simulink model "TCPZybo"  (Simulink 8.3)
settings: Solver=FixedStepDiscrete  StartTime=0.0  StopTime=inf  FixedStep=0.5  RelTol=1e-3
StartFcn:
  | localAddEventListener
libraries: simulink x5, hdlsllib x2, instrumentlib x2
settings Model: xpc_rtwmakecfg_data=_xpcetherlib__xpcether8255xlib__xpcetherGbElib__xpcnblib_  Creator=laca  LastModifiedBy=laca
settings OptimizationCC: BlockReduction=off
settings DebuggingCC: UnderspecifiedInitializationDetection=Simplified  MultiTaskDSMMsg=warning  MultiTaskCondExecSysMsg=none  StateNameClashWarn=none
settings RTWCC: IncludeERTFirstTime=on
settings GRTTargetCC: CombineOutputUpdateFcns=on  GRTInterface=off

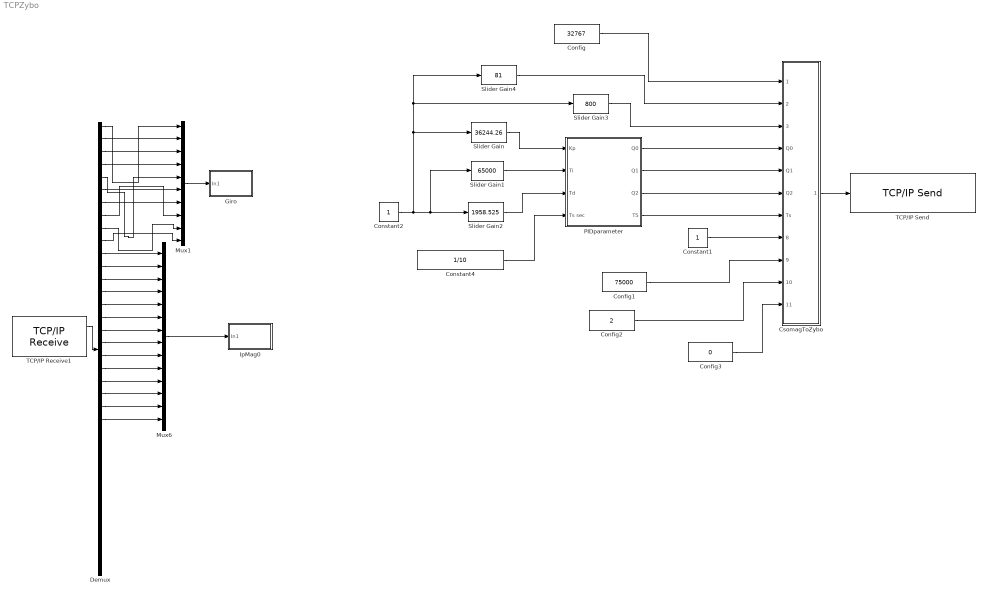
== system TCPZybo ==
  Config : Constant  Value=32767
  Config1 : Constant  Value=75000
  Config2 : Constant  Value=2
  Config3 : Constant  Value=0
  Constant1 : Constant
  Constant2 : Constant
  Constant4 : Constant  Value=1/10
  CsomagToZybo : Subsystem
  Demux : Demux  Outputs=36
  Giro : Subsystem
  IpMag0 : Subsystem
  Mux1 : Mux  Inputs=10
  Mux6 : Mux  Inputs=14
  PIDparameter : Subsystem
  Slider Gain : simulink/Math Operations/Slider Gain  low=0  gain=36244.26  high=65000
  Slider Gain1 : simulink/Math Operations/Slider Gain  low=0  gain=65000  high=65000
  Slider Gain2 : simulink/Math Operations/Slider Gain  low=0  gain=1958.525  high=5000
  Slider Gain3 : simulink/Math Operations/Slider Gain  low=-10000  gain=800  high=10000
  Slider Gain4 : simulink/Math Operations/Slider Gain  low=-180  gain=81  high=180
  TCP/IP Receive1 : instrumentlib/TCP//IP Receive  Host=192.168.0.10  Port=7  DataSize="[1  36]"  EnableBlockingMode=off  Timeout=100  SampleTime=1  DataType=int16  ByteOrder=LittleEndian
  TCP/IP Send : instrumentlib/TCP//IP Send  Host=192.168.0.10  Port=7  EnableBlockingMode=off  Timeout=10  ByteOrder=LittleEndian
  wires:
  Demux/1 -> Mux1/1
  Demux/2 -> Mux1/2
  Demux/3 -> Mux1/3
  TCP/IP Receive1/1 -> Demux/1
  Demux/11 -> Mux6/1
  Demux/24 -> Mux6/14
  Demux/23 -> Mux6/13
  Demux/22 -> Mux6/12
  Demux/21 -> Mux6/11
  Demux/20 -> Mux6/10
  Demux/19 -> Mux6/9
  Demux/18 -> Mux6/8
  Demux/17 -> Mux6/7
  Demux/16 -> Mux6/6
  Demux/15 -> Mux6/5
  Demux/14 -> Mux6/4
  Demux/13 -> Mux6/3
  Demux/12 -> Mux6/2
  Mux6/1 -> IpMag0/1(In1)
  Demux/10 -> Mux1/10
  Demux/9 -> Mux1/9
  Demux/8 -> Mux1/8
  Demux/7 -> Mux1/7
  Demux/6 -> Mux1/6
  Demux/5 -> Mux1/5
  Demux/4 -> Mux1/4
  Mux1/1 -> Giro/1(In1)
  CsomagToZybo/1(Out1) -> TCP/IP Send/1
  Constant2/1 -> Slider Gain4/1, Slider Gain3/1, Slider Gain/1, Slider Gain1/1, Slider Gain2/1
  Slider Gain/1 -> PIDparameter/1(Kp)
  Slider Gain1/1 -> PIDparameter/2(Ti)
  Slider Gain2/1 -> PIDparameter/3(Td)
  Constant4/1 -> PIDparameter/4(Ts sec)
  PIDparameter/4(TS) -> CsomagToZybo/7(Ts)
  PIDparameter/3(Q2) -> CsomagToZybo/6(Q2)
  PIDparameter/2(Q1) -> CsomagToZybo/5(Q1)
  PIDparameter/1(Q0) -> CsomagToZybo/4(Q0)
  Slider Gain3/1 -> CsomagToZybo/3(RefSpeed)
  Slider Gain4/1 -> CsomagToZybo/2(RefPos)
  Config/1 -> CsomagToZybo/1(Config)
  Constant1/1 -> CsomagToZybo/8(Egyeb)
  Config1/1 -> CsomagToZybo/9(PwmFrek)
  Config2/1 -> CsomagToZybo/10(qSav)
  Config3/1 -> CsomagToZybo/11(SugaeakAranya)

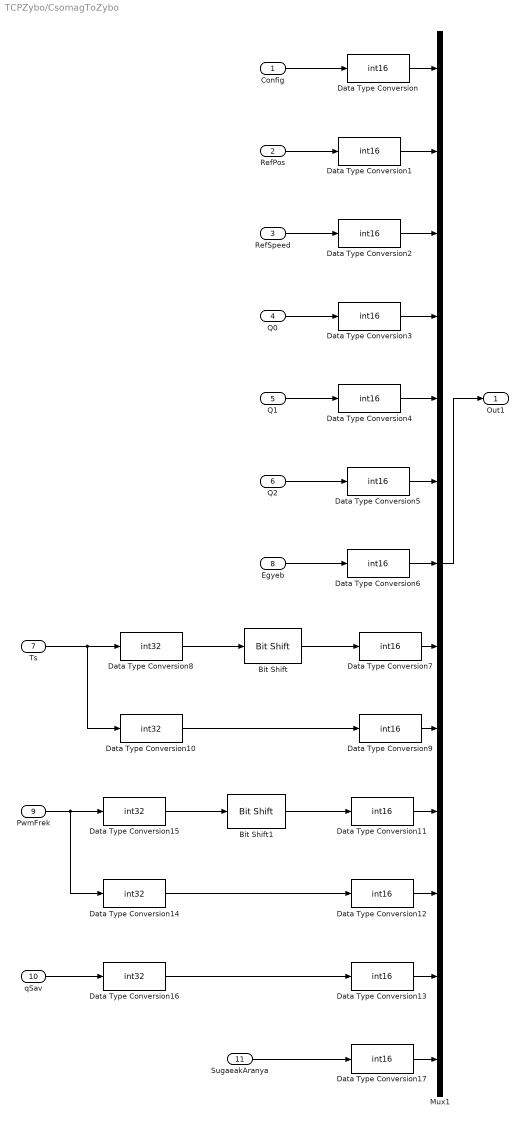
== system TCPZybo/CsomagToZybo ==
  Config : Inport
  RefPos : Inport  Port=2
  RefSpeed : Inport  Port=3
  Q0 : Inport  Port=4
  Q1 : Inport  Port=5
  Q2 : Inport  Port=6
  Ts : Inport  Port=7
  Egyeb : Inport  Port=8
  PwmFrek : Inport  Port=9
  qSav : Inport  Port=10
  SugaeakAranya : Inport  Port=11
  Bit Shift : hdlsllib/HDL Operations/Bit Shift  mode=Shift Right Arithmetic  N=16
  Bit Shift1 : hdlsllib/HDL Operations/Bit Shift  mode=Shift Right Arithmetic  N=16
  Data Type Conversion{,1..7,9,11..13,17} (13 alike) : DataTypeConversion  OutDataTypeStr=int16
  Data Type Conversion{8,10,14..16} (5 alike) : DataTypeConversion  OutDataTypeStr=int32
  Mux1 : Mux  Inputs=13
  Out1 : Outport
  wires:
  Mux1/1 -> Out1/1
  Data Type Conversion/1 -> Mux1/1
  Data Type Conversion1/1 -> Mux1/2
  Data Type Conversion2/1 -> Mux1/3
  Data Type Conversion3/1 -> Mux1/4
  Data Type Conversion4/1 -> Mux1/5
  Data Type Conversion5/1 -> Mux1/6
  Data Type Conversion6/1 -> Mux1/7
  Config/1 -> Data Type Conversion/1
  RefPos/1 -> Data Type Conversion1/1
  RefSpeed/1 -> Data Type Conversion2/1
  Q0/1 -> Data Type Conversion3/1
  Q1/1 -> Data Type Conversion4/1
  Q2/1 -> Data Type Conversion5/1
  Egyeb/1 -> Data Type Conversion6/1
  Ts/1 -> Data Type Conversion10/1, Data Type Conversion8/1
  Data Type Conversion10/1 -> Data Type Conversion9/1
  Data Type Conversion7/1 -> Mux1/8
  Data Type Conversion9/1 -> Mux1/9
  Data Type Conversion8/1 -> Bit Shift/1
  Bit Shift/1 -> Data Type Conversion7/1
  Data Type Conversion11/1 -> Mux1/10
  Data Type Conversion12/1 -> Mux1/11
  Data Type Conversion13/1 -> Mux1/12
  PwmFrek/1 -> Data Type Conversion14/1, Data Type Conversion15/1
  Data Type Conversion14/1 -> Data Type Conversion12/1
  Data Type Conversion15/1 -> Bit Shift1/1
  Bit Shift1/1 -> Data Type Conversion11/1
  Data Type Conversion16/1 -> Data Type Conversion13/1
  qSav/1 -> Data Type Conversion16/1
  Data Type Conversion17/1 -> Mux1/13
  SugaeakAranya/1 -> Data Type Conversion17/1

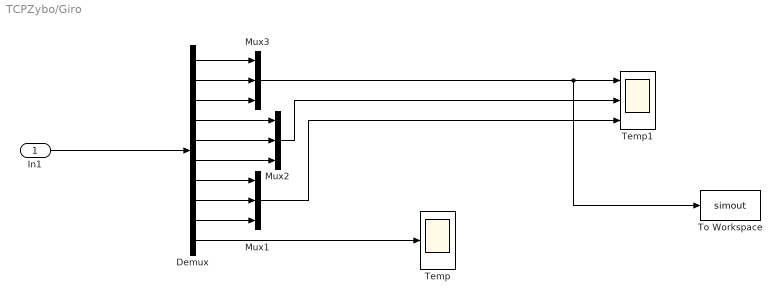
== system TCPZybo/Giro ==
  In1 : Inport
  Demux : Demux  Outputs=10
  Mux1 : Mux  Inputs=3
  Mux2 : Mux  Inputs=3
  Mux3 : Mux  Inputs=3
  Temp : Scope
      settings: TickLabels=on  TimeRange=2000  YMin=204.25  YMax=225.75  SaveName=ScopeData4  SampleInput=on
  Temp1 : Scope  NumInputPorts=3
      settings: TickLabels=on  TimeRange=2000  YMin=204.25~-5~-5  YMax=225.75~5~5  SaveName=ScopeData2  SampleInput=on
  To Workspace : ToWorkspace  VariableName=simout  SaveFormat=Structure With Time  SampleTime=-1
  wires:
  In1/1 -> Demux/1
  Demux/1 -> Mux3/1
  Demux/2 -> Mux3/2
  Demux/3 -> Mux3/3
  Demux/4 -> Mux2/1
  Demux/5 -> Mux2/2
  Demux/6 -> Mux2/3
  Demux/7 -> Mux1/1
  Demux/8 -> Mux1/2
  Demux/9 -> Mux1/3
  Mux3/1 -> Temp1/1, To Workspace/1
  Mux2/1 -> Temp1/2
  Mux1/1 -> Temp1/3
  Demux/10 -> Temp/1

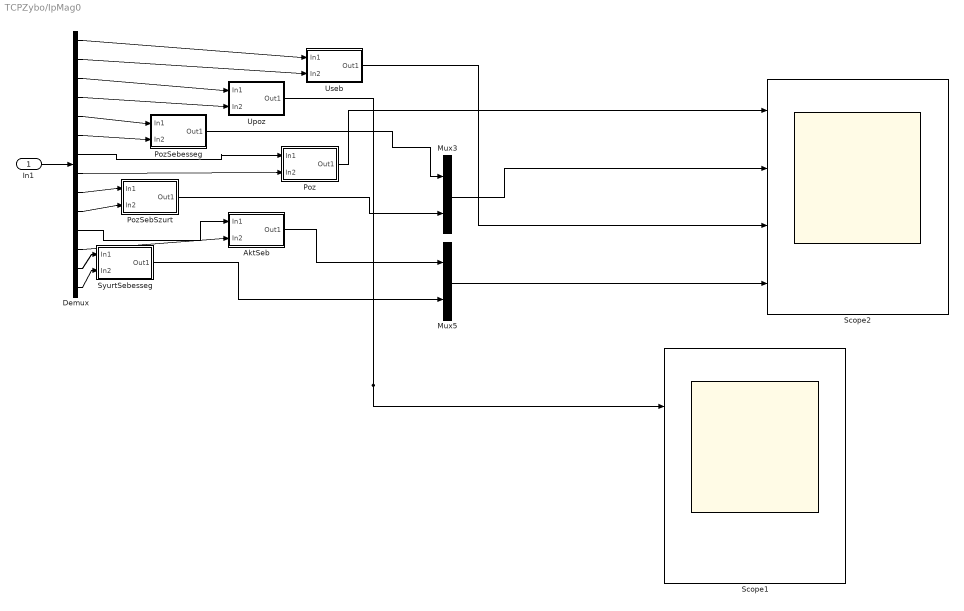
== system TCPZybo/IpMag0 ==
  In1 : Inport
  AktSeb : Subsystem
  Demux : Demux  Outputs=14
  Mux3 : Mux  Inputs=2
  Mux5 : Mux  Inputs=2
  Poz : Subsystem
  PozSebSzurt : Subsystem
  PozSebesseg : Subsystem
  Scope1 : Scope  NumInputPorts=2
      settings: TickLabels=on  TimeRange=2000  YMin=-68250~-1  YMax=-61750~1  SampleInput=on
  Scope2 : Scope  NumInputPorts=4
      settings: TickLabels=on  TimeRange=2000  YMin=-10500~-80~-1~-1  YMax=-7750~50~-1~1  SaveName=ScopeData3  SampleInput=on
  SyurtSebesseg : Subsystem
  Upoz : Subsystem
  Useb : Subsystem
  wires:
  Demux/5 -> PozSebesseg/1(In1)
  Demux/6 -> PozSebesseg/2(In2)
  Demux/4 -> Upoz/2(In2)
  Demux/3 -> Upoz/1(In1)
  Demux/11 -> AktSeb/1(In1)
  Demux/12 -> AktSeb/2(In2)
  Demux/13 -> SyurtSebesseg/1(In1)
  Demux/14 -> SyurtSebesseg/2(In2)
  PozSebesseg/1(Out1) -> Mux3/1
  PozSebSzurt/1(Out1) -> Mux3/2
  AktSeb/1(Out1) -> Mux5/1
  SyurtSebesseg/1(Out1) -> Mux5/2
  Poz/1(Out1) -> Scope2/1
  Mux3/1 -> Scope2/2
  Mux5/1 -> Scope2/4
  In1/1 -> Demux/1
  Demux/7 -> Poz/1(In1)
  Demux/8 -> Poz/2(In2)
  Demux/9 -> PozSebSzurt/1(In1)
  Demux/10 -> PozSebSzurt/2(In2)
  Useb/1(Out1) -> Scope2/3
  Upoz/1(Out1) -> Scope1/1
  ? -> Scope1/2
  Demux/1 -> Useb/1(In1)
  Demux/2 -> Useb/2(In2)

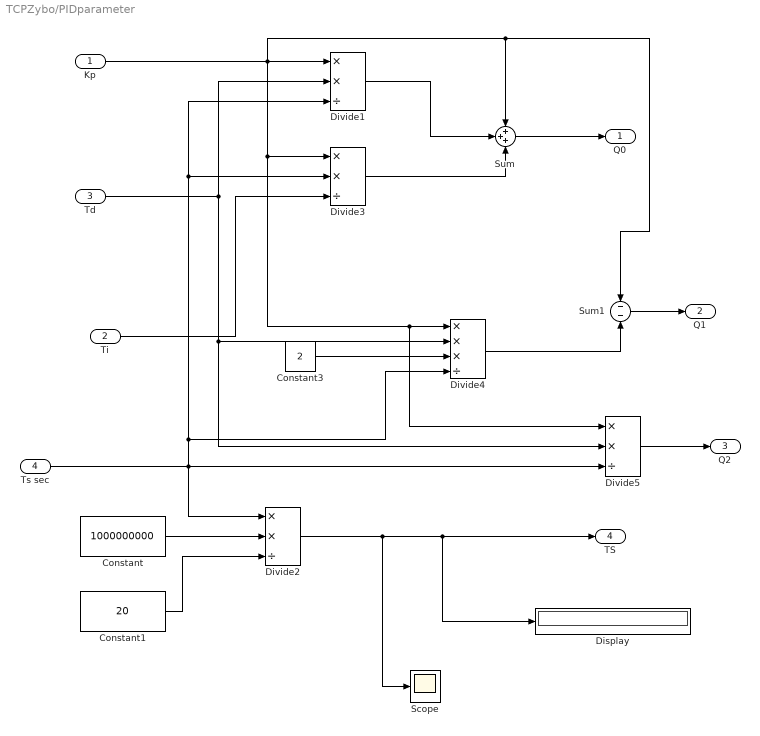
== system TCPZybo/PIDparameter ==
  Kp : Inport
  Ti : Inport  Port=2
  Td : Inport  Port=3
  Ts sec : Inport  Port=4
  Constant : Constant  Value=1000000000
  Constant1 : Constant  Value=20
  Constant3 : Constant  Value=2
  Display : Display
  Divide{1..3,5} (4 alike) : Product  Inputs=**/
  Divide4 : Product  Inputs=***/
  Scope : Scope
  Sum : Sum  Inputs=+++
  Sum1 : Sum  Inputs=--
  Q0 : Outport
  Q1 : Outport  Port=2
  Q2 : Outport  Port=3
  TS : Outport  Port=4
  wires:
  Divide2/1 -> Scope/1, Display/1, TS/1
  Ts sec/1 -> Divide5/3, Divide2/1, Divide4/4, Divide3/2, Divide1/3
  Constant/1 -> Divide2/2
  Constant1/1 -> Divide2/3
  Ti/1 -> Divide3/3
  Td/1 -> Divide1/2, Divide5/2, Divide4/2
  Divide3/1 -> Sum/3
  Divide1/1 -> Sum/2
  Kp/1 -> Sum1/1, Sum/1, Divide5/1, Divide4/1, Divide3/1, Divide1/1
  Sum/1 -> Q0/1
  Constant3/1 -> Divide4/3
  Divide4/1 -> Sum1/2
  Sum1/1 -> Q1/1
  Divide5/1 -> Q2/1

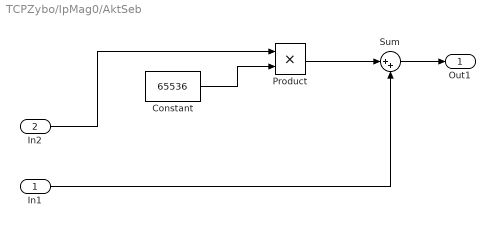
== system TCPZybo/IpMag0/AktSeb ==
  In1 : Inport
  In2 : Inport  Port=2
  Constant : Constant  Value=65536
  Product : Product
  Sum : Sum  Inputs=|++
  Out1 : Outport
  wires:
  Sum/1 -> Out1/1
  Product/1 -> Sum/1
  Constant/1 -> Product/2
  In2/1 -> Product/1
  In1/1 -> Sum/2

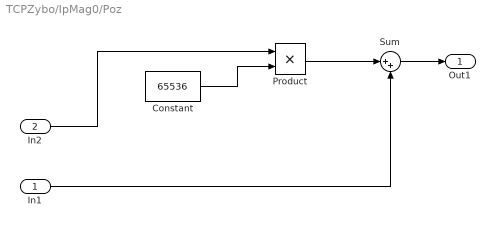
== system TCPZybo/IpMag0/Poz ==
  In1 : Inport
  In2 : Inport  Port=2
  Constant : Constant  Value=65536
  Product : Product
  Sum : Sum  Inputs=|++
  Out1 : Outport
  wires:
  Sum/1 -> Out1/1
  Product/1 -> Sum/1
  Constant/1 -> Product/2
  In2/1 -> Product/1
  In1/1 -> Sum/2

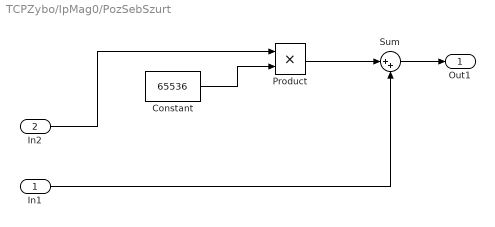
== system TCPZybo/IpMag0/PozSebSzurt ==
  In1 : Inport
  In2 : Inport  Port=2
  Constant : Constant  Value=65536
  Product : Product
  Sum : Sum  Inputs=|++
  Out1 : Outport
  wires:
  Sum/1 -> Out1/1
  Product/1 -> Sum/1
  Constant/1 -> Product/2
  In2/1 -> Product/1
  In1/1 -> Sum/2

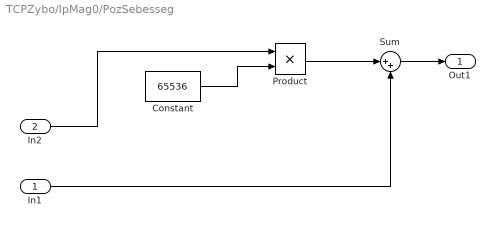
== system TCPZybo/IpMag0/PozSebesseg ==
  In1 : Inport
  In2 : Inport  Port=2
  Constant : Constant  Value=65536
  Product : Product
  Sum : Sum  Inputs=|++
  Out1 : Outport
  wires:
  Sum/1 -> Out1/1
  Product/1 -> Sum/1
  Constant/1 -> Product/2
  In2/1 -> Product/1
  In1/1 -> Sum/2

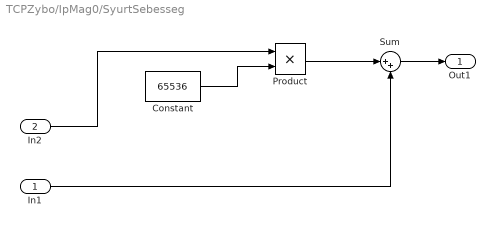
== system TCPZybo/IpMag0/SyurtSebesseg ==
  In1 : Inport
  In2 : Inport  Port=2
  Constant : Constant  Value=65536
  Product : Product
  Sum : Sum  Inputs=|++
  Out1 : Outport
  wires:
  Sum/1 -> Out1/1
  Product/1 -> Sum/1
  Constant/1 -> Product/2
  In2/1 -> Product/1
  In1/1 -> Sum/2

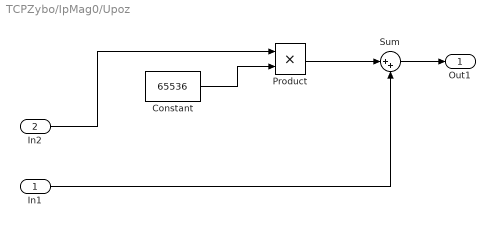
== system TCPZybo/IpMag0/Upoz ==
  In1 : Inport
  In2 : Inport  Port=2
  Constant : Constant  Value=65536
  Product : Product
  Sum : Sum  Inputs=|++
  Out1 : Outport
  wires:
  Sum/1 -> Out1/1
  Product/1 -> Sum/1
  Constant/1 -> Product/2
  In2/1 -> Product/1
  In1/1 -> Sum/2

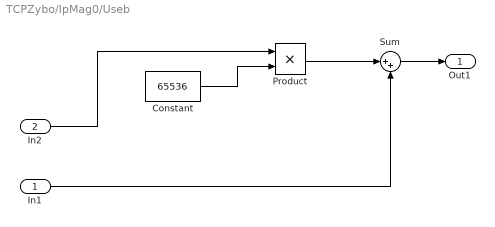
== system TCPZybo/IpMag0/Useb ==
  In1 : Inport
  In2 : Inport  Port=2
  Constant : Constant  Value=65536
  Product : Product
  Sum : Sum  Inputs=|++
  Out1 : Outport
  wires:
  Sum/1 -> Out1/1
  Product/1 -> Sum/1
  Constant/1 -> Product/2
  In2/1 -> Product/1
  In1/1 -> Sum/2
